simulink library "CRYP_OLSERVO"  (Simulink 8.6)
settings: Solver=VariableStepAuto  StartTime=0.0  StopTime=10.0  RelTol=1e-3
libraries: cdsTP x48, cdsEpicsOut x48, cdsFiltCtrl x25, cdsEpicsStringIn x24, cdsRms x24, cdsFilt x24, cdsMuxMatrix x2, lockin x1
(part 2 of 4)

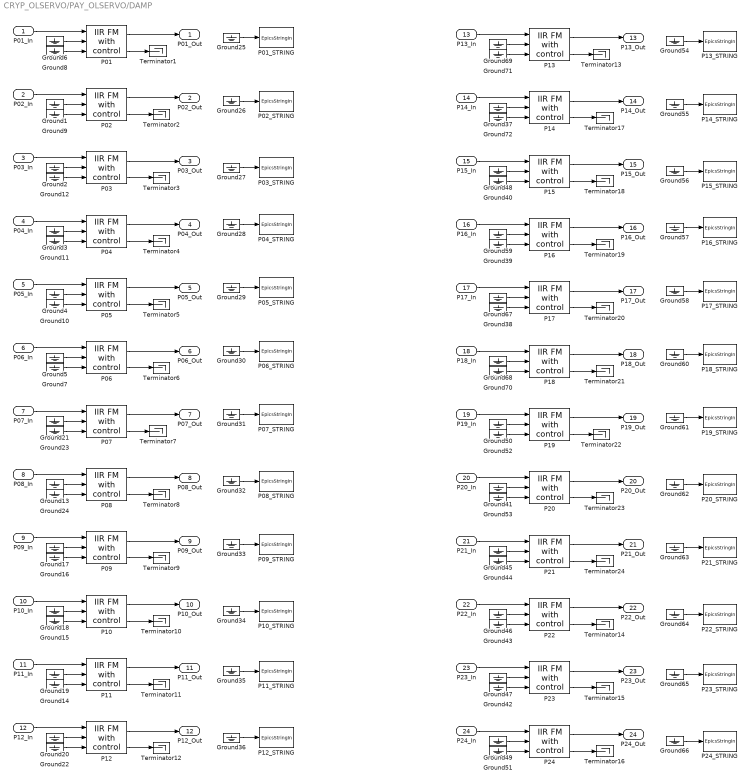
== system CRYP_OLSERVO/PAY_OLSERVO/DAMP ==
  P01_In : Inport
  P02_In : Inport  Port=2
  P03_In : Inport  Port=3
  P04_In : Inport  Port=4
  P05_In : Inport  Port=5
  P06_In : Inport  Port=6
  P07_In : Inport  Port=7
  P08_In : Inport  Port=8
  P09_In : Inport  Port=9
  P10_In : Inport  Port=10
  P11_In : Inport  Port=11
  P12_In : Inport  Port=12
  P13_In : Inport  Port=13
  P14_In : Inport  Port=14
  P15_In : Inport  Port=15
  P16_In : Inport  Port=16
  P17_In : Inport  Port=17
  P18_In : Inport  Port=18
  P19_In : Inport  Port=19
  P20_In : Inport  Port=20
  P21_In : Inport  Port=21
  P22_In : Inport  Port=22
  P23_In : Inport  Port=23
  P24_In : Inport  Port=24
  Ground{1..72} (72 alike) : Ground
  P01 : cdsFiltCtrl/IIR FM with control  Tag=cdsFiltCtrl  Description=|
      | cdsFiltCntrl is the standard IIR filter module (exactly the same as cdsFilt) but with added control data output 'Ctrl'. Filter module digital signal output appears on the first output, which is called 'Val'. 'Ctrl' output has a bit pattern encoding the state of filter's on/off switches (FM1 through FM10). The bit values are:
      |                                                                                                                                                                                                                                                                                                                                       
      | module 	hex	dec                                                                                                                                                                                                                                                                                                                       
      | -----------------------                                                                                                                                                                                                                                                                                                               
      | FM1	0x20                    32                                                                                                                                                                                                                                                                                                        
      | FM2	0x80                     128                                                                                                                                                                                                                                                                                                      
      | FM3	0x200                   512                                                                                                                                                                                                                                                                                                       
      | FM4	0x800                   2048                                                                                                                                                                                                                                                                                                      
      | FM5	0x2000                 8192                                                                                                                                                                                                                                                                                                       
      | FM6	0x8000                 32768                                                                                                                                                                                                                                                                                                      
      | FM7	0x20000                131072                                                                                                                                                                                                                                                                                                     
      | FM8	0x80000                 524288                                                                                                                                                                                                                                                                                                    
      | FM9	0x200000               2097152                                                                                                                                                                                                                                                                                                    
      | FM10	0x800000               8388608                                                                                                                                                                                                                                                                                                   
      |                                                                                                                                                                                                                                                                                                                                       
      | This bit data can be used to drive some other switches or it can be output using a binary I/O module.
      settings: AttributesFormatString=%<Tag>
  P01_STRING : cdsEpicsStringIn/EpicsStringIn  Tag=cdsEpicsStringIn  Description=cdsEpicsStringIn
      settings: AttributesFormatString=%<Tag>
  P02 : cdsFiltCtrl/IIR FM with control  Tag=cdsFiltCtrl  Description=|
      | cdsFiltCntrl is the standard IIR filter module (exactly the same as cdsFilt) but with added control data output 'Ctrl'. Filter module digital signal output appears on the first output, which is called 'Val'. 'Ctrl' output has a bit pattern encoding the state of filter's on/off switches (FM1 through FM10). The bit values are:
      |                                                                                                                                                                                                                                                                                                                                       
      | module 	hex	dec                                                                                                                                                                                                                                                                                                                       
      | -----------------------                                                                                                                                                                                                                                                                                                               
      | FM1	0x20                    32                                                                                                                                                                                                                                                                                                        
      | FM2	0x80                     128                                                                                                                                                                                                                                                                                                      
      | FM3	0x200                   512                                                                                                                                                                                                                                                                                                       
      | FM4	0x800                   2048                                                                                                                                                                                                                                                                                                      
      | FM5	0x2000                 8192                                                                                                                                                                                                                                                                                                       
      | FM6	0x8000                 32768                                                                                                                                                                                                                                                                                                      
      | FM7	0x20000                131072                                                                                                                                                                                                                                                                                                     
      | FM8	0x80000                 524288                                                                                                                                                                                                                                                                                                    
      | FM9	0x200000               2097152                                                                                                                                                                                                                                                                                                    
      | FM10	0x800000               8388608                                                                                                                                                                                                                                                                                                   
      |                                                                                                                                                                                                                                                                                                                                       
      | This bit data can be used to drive some other switches or it can be output using a binary I/O module.
      settings: AttributesFormatString=%<Tag>
  P02_STRING : cdsEpicsStringIn/EpicsStringIn  Tag=cdsEpicsStringIn  Description=cdsEpicsStringIn
      settings: AttributesFormatString=%<Tag>
  P03 : cdsFiltCtrl/IIR FM with control  Tag=cdsFiltCtrl  Description=|
      | cdsFiltCntrl is the standard IIR filter module (exactly the same as cdsFilt) but with added control data output 'Ctrl'. Filter module digital signal output appears on the first output, which is called 'Val'. 'Ctrl' output has a bit pattern encoding the state of filter's on/off switches (FM1 through FM10). The bit values are:
      |                                                                                                                                                                                                                                                                                                                                       
      | module 	hex	dec                                                                                                                                                                                                                                                                                                                       
      | -----------------------                                                                                                                                                                                                                                                                                                               
      | FM1	0x20                    32                                                                                                                                                                                                                                                                                                        
      | FM2	0x80                     128                                                                                                                                                                                                                                                                                                      
      | FM3	0x200                   512                                                                                                                                                                                                                                                                                                       
      | FM4	0x800                   2048                                                                                                                                                                                                                                                                                                      
      | FM5	0x2000                 8192                                                                                                                                                                                                                                                                                                       
      | FM6	0x8000                 32768                                                                                                                                                                                                                                                                                                      
      | FM7	0x20000                131072                                                                                                                                                                                                                                                                                                     
      | FM8	0x80000                 524288                                                                                                                                                                                                                                                                                                    
      | FM9	0x200000               2097152                                                                                                                                                                                                                                                                                                    
      | FM10	0x800000               8388608                                                                                                                                                                                                                                                                                                   
      |                                                                                                                                                                                                                                                                                                                                       
      | This bit data can be used to drive some other switches or it can be output using a binary I/O module.
      settings: AttributesFormatString=%<Tag>
  P03_STRING : cdsEpicsStringIn/EpicsStringIn  Tag=cdsEpicsStringIn  Description=cdsEpicsStringIn
      settings: AttributesFormatString=%<Tag>
  P04 : cdsFiltCtrl/IIR FM with control  Tag=cdsFiltCtrl  Description=|
      | cdsFiltCntrl is the standard IIR filter module (exactly the same as cdsFilt) but with added control data output 'Ctrl'. Filter module digital signal output appears on the first output, which is called 'Val'. 'Ctrl' output has a bit pattern encoding the state of filter's on/off switches (FM1 through FM10). The bit values are:
      |                                                                                                                                                                                                                                                                                                                                       
      | module 	hex	dec                                                                                                                                                                                                                                                                                                                       
      | -----------------------                                                                                                                                                                                                                                                                                                               
      | FM1	0x20                    32                                                                                                                                                                                                                                                                                                        
      | FM2	0x80                     128                                                                                                                                                                                                                                                                                                      
      | FM3	0x200                   512                                                                                                                                                                                                                                                                                                       
      | FM4	0x800                   2048                                                                                                                                                                                                                                                                                                      
      | FM5	0x2000                 8192                                                                                                                                                                                                                                                                                                       
      | FM6	0x8000                 32768                                                                                                                                                                                                                                                                                                      
      | FM7	0x20000                131072                                                                                                                                                                                                                                                                                                     
      | FM8	0x80000                 524288                                                                                                                                                                                                                                                                                                    
      | FM9	0x200000               2097152                                                                                                                                                                                                                                                                                                    
      | FM10	0x800000               8388608                                                                                                                                                                                                                                                                                                   
      |                                                                                                                                                                                                                                                                                                                                       
      | This bit data can be used to drive some other switches or it can be output using a binary I/O module.
      settings: AttributesFormatString=%<Tag>
  P04_STRING : cdsEpicsStringIn/EpicsStringIn  Tag=cdsEpicsStringIn  Description=cdsEpicsStringIn
      settings: AttributesFormatString=%<Tag>
  P05 : cdsFiltCtrl/IIR FM with control  Tag=cdsFiltCtrl  Description=|
      | cdsFiltCntrl is the standard IIR filter module (exactly the same as cdsFilt) but with added control data output 'Ctrl'. Filter module digital signal output appears on the first output, which is called 'Val'. 'Ctrl' output has a bit pattern encoding the state of filter's on/off switches (FM1 through FM10). The bit values are:
      |                                                                                                                                                                                                                                                                                                                                       
      | module 	hex	dec                                                                                                                                                                                                                                                                                                                       
      | -----------------------                                                                                                                                                                                                                                                                                                               
      | FM1	0x20                    32                                                                                                                                                                                                                                                                                                        
      | FM2	0x80                     128                                                                                                                                                                                                                                                                                                      
      | FM3	0x200                   512                                                                                                                                                                                                                                                                                                       
      | FM4	0x800                   2048                                                                                                                                                                                                                                                                                                      
      | FM5	0x2000                 8192                                                                                                                                                                                                                                                                                                       
      | FM6	0x8000                 32768                                                                                                                                                                                                                                                                                                      
      | FM7	0x20000                131072                                                                                                                                                                                                                                                                                                     
      | FM8	0x80000                 524288                                                                                                                                                                                                                                                                                                    
      | FM9	0x200000               2097152                                                                                                                                                                                                                                                                                                    
      | FM10	0x800000               8388608                                                                                                                                                                                                                                                                                                   
      |                                                                                                                                                                                                                                                                                                                                       
      | This bit data can be used to drive some other switches or it can be output using a binary I/O module.
      settings: AttributesFormatString=%<Tag>
  P05_STRING : cdsEpicsStringIn/EpicsStringIn  Tag=cdsEpicsStringIn  Description=cdsEpicsStringIn
      settings: AttributesFormatString=%<Tag>
  P06 : cdsFiltCtrl/IIR FM with control  Tag=cdsFiltCtrl  Description=|
      | cdsFiltCntrl is the standard IIR filter module (exactly the same as cdsFilt) but with added control data output 'Ctrl'. Filter module digital signal output appears on the first output, which is called 'Val'. 'Ctrl' output has a bit pattern encoding the state of filter's on/off switches (FM1 through FM10). The bit values are:
      |                                                                                                                                                                                                                                                                                                                                       
      | module 	hex	dec                                                                                                                                                                                                                                                                                                                       
      | -----------------------                                                                                                                                                                                                                                                                                                               
      | FM1	0x20                    32                                                                                                                                                                                                                                                                                                        
      | FM2	0x80                     128                                                                                                                                                                                                                                                                                                      
      | FM3	0x200                   512                                                                                                                                                                                                                                                                                                       
      | FM4	0x800                   2048                                                                                                                                                                                                                                                                                                      
      | FM5	0x2000                 8192                                                                                                                                                                                                                                                                                                       
      | FM6	0x8000                 32768                                                                                                                                                                                                                                                                                                      
      | FM7	0x20000                131072                                                                                                                                                                                                                                                                                                     
      | FM8	0x80000                 524288                                                                                                                                                                                                                                                                                                    
      | FM9	0x200000               2097152                                                                                                                                                                                                                                                                                                    
      | FM10	0x800000               8388608                                                                                                                                                                                                                                                                                                   
      |                                                                                                                                                                                                                                                                                                                                       
      | This bit data can be used to drive some other switches or it can be output using a binary I/O module.
      settings: AttributesFormatString=%<Tag>
  P06_STRING : cdsEpicsStringIn/EpicsStringIn  Tag=cdsEpicsStringIn  Description=cdsEpicsStringIn
      settings: AttributesFormatString=%<Tag>
  P07 : cdsFiltCtrl/IIR FM with control  Tag=cdsFiltCtrl  Description=|
      | cdsFiltCntrl is the standard IIR filter module (exactly the same as cdsFilt) but with added control data output 'Ctrl'. Filter module digital signal output appears on the first output, which is called 'Val'. 'Ctrl' output has a bit pattern encoding the state of filter's on/off switches (FM1 through FM10). The bit values are:
      |                                                                                                                                                                                                                                                                                                                                       
      | module 	hex	dec                                                                                                                                                                                                                                                                                                                       
      | -----------------------                                                                                                                                                                                                                                                                                                               
      | FM1	0x20                    32                                                                                                                                                                                                                                                                                                        
      | FM2	0x80                     128                                                                                                                                                                                                                                                                                                      
      | FM3	0x200                   512                                                                                                                                                                                                                                                                                                       
      | FM4	0x800                   2048                                                                                                                                                                                                                                                                                                      
      | FM5	0x2000                 8192                                                                                                                                                                                                                                                                                                       
      | FM6	0x8000                 32768                                                                                                                                                                                                                                                                                                      
      | FM7	0x20000                131072                                                                                                                                                                                                                                                                                                     
      | FM8	0x80000                 524288                                                                                                                                                                                                                                                                                                    
      | FM9	0x200000               2097152                                                                                                                                                                                                                                                                                                    
      | FM10	0x800000               8388608                                                                                                                                                                                                                                                                                                   
      |                                                                                                                                                                                                                                                                                                                                       
      | This bit data can be used to drive some other switches or it can be output using a binary I/O module.
      settings: AttributesFormatString=%<Tag>
  P07_STRING : cdsEpicsStringIn/EpicsStringIn  Tag=cdsEpicsStringIn  Description=cdsEpicsStringIn
      settings: AttributesFormatString=%<Tag>
  P08 : cdsFiltCtrl/IIR FM with control  Tag=cdsFiltCtrl  Description=|
      | cdsFiltCntrl is the standard IIR filter module (exactly the same as cdsFilt) but with added control data output 'Ctrl'. Filter module digital signal output appears on the first output, which is called 'Val'. 'Ctrl' output has a bit pattern encoding the state of filter's on/off switches (FM1 through FM10). The bit values are:
      |                                                                                                                                                                                                                                                                                                                                       
      | module 	hex	dec                                                                                                                                                                                                                                                                                                                       
      | -----------------------                                                                                                                                                                                                                                                                                                               
      | FM1	0x20                    32                                                                                                                                                                                                                                                                                                        
      | FM2	0x80                     128                                                                                                                                                                                                                                                                                                      
      | FM3	0x200                   512                                                                                                                                                                                                                                                                                                       
      | FM4	0x800                   2048                                                                                                                                                                                                                                                                                                      
      | FM5	0x2000                 8192                                                                                                                                                                                                                                                                                                       
      | FM6	0x8000                 32768                                                                                                                                                                                                                                                                                                      
      | FM7	0x20000                131072                                                                                                                                                                                                                                                                                                     
      | FM8	0x80000                 524288                                                                                                                                                                                                                                                                                                    
      | FM9	0x200000               2097152                                                                                                                                                                                                                                                                                                    
      | FM10	0x800000               8388608                                                                                                                                                                                                                                                                                                   
      |                                                                                                                                                                                                                                                                                                                                       
      | This bit data can be used to drive some other switches or it can be output using a binary I/O module.
      settings: AttributesFormatString=%<Tag>
  P08_STRING : cdsEpicsStringIn/EpicsStringIn  Tag=cdsEpicsStringIn  Description=cdsEpicsStringIn
      settings: AttributesFormatString=%<Tag>
  P09 : cdsFiltCtrl/IIR FM with control  Tag=cdsFiltCtrl  Description=|
      | cdsFiltCntrl is the standard IIR filter module (exactly the same as cdsFilt) but with added control data output 'Ctrl'. Filter module digital signal output appears on the first output, which is called 'Val'. 'Ctrl' output has a bit pattern encoding the state of filter's on/off switches (FM1 through FM10). The bit values are:
      |                                                                                                                                                                                                                                                                                                                                       
      | module 	hex	dec                                                                                                                                                                                                                                                                                                                       
      | -----------------------                                                                                                                                                                                                                                                                                                               
      | FM1	0x20                    32                                                                                                                                                                                                                                                                                                        
      | FM2	0x80                     128                                                                                                                                                                                                                                                                                                      
      | FM3	0x200                   512                                                                                                                                                                                                                                                                                                       
      | FM4	0x800                   2048                                                                                                                                                                                                                                                                                                      
      | FM5	0x2000                 8192                                                                                                                                                                                                                                                                                                       
      | FM6	0x8000                 32768                                                                                                                                                                                                                                                                                                      
      | FM7	0x20000                131072                                                                                                                                                                                                                                                                                                     
      | FM8	0x80000                 524288                                                                                                                                                                                                                                                                                                    
      | FM9	0x200000               2097152                                                                                                                                                                                                                                                                                                    
      | FM10	0x800000               8388608                                                                                                                                                                                                                                                                                                   
      |                                                                                                                                                                                                                                                                                                                                       
      | This bit data can be used to drive some other switches or it can be output using a binary I/O module.
      settings: AttributesFormatString=%<Tag>
  P09_STRING : cdsEpicsStringIn/EpicsStringIn  Tag=cdsEpicsStringIn  Description=cdsEpicsStringIn
      settings: AttributesFormatString=%<Tag>
  P10 : cdsFiltCtrl/IIR FM with control  Tag=cdsFiltCtrl  Description=|
      | cdsFiltCntrl is the standard IIR filter module (exactly the same as cdsFilt) but with added control data output 'Ctrl'. Filter module digital signal output appears on the first output, which is called 'Val'. 'Ctrl' output has a bit pattern encoding the state of filter's on/off switches (FM1 through FM10). The bit values are:
      |                                                                                                                                                                                                                                                                                                                                       
      | module 	hex	dec                                                                                                                                                                                                                                                                                                                       
      | -----------------------                                                                                                                                                                                                                                                                                                               
      | FM1	0x20                    32                                                                                                                                                                                                                                                                                                        
      | FM2	0x80                     128                                                                                                                                                                                                                                                                                                      
      | FM3	0x200                   512                                                                                                                                                                                                                                                                                                       
      | FM4	0x800                   2048                                                                                                                                                                                                                                                                                                      
      | FM5	0x2000                 8192                                                                                                                                                                                                                                                                                                       
      | FM6	0x8000                 32768                                                                                                                                                                                                                                                                                                      
      | FM7	0x20000                131072                                                                                                                                                                                                                                                                                                     
      | FM8	0x80000                 524288                                                                                                                                                                                                                                                                                                    
      | FM9	0x200000               2097152                                                                                                                                                                                                                                                                                                    
      | FM10	0x800000               8388608                                                                                                                                                                                                                                                                                                   
      |                                                                                                                                                                                                                                                                                                                                       
      | This bit data can be used to drive some other switches or it can be output using a binary I/O module.
      settings: AttributesFormatString=%<Tag>
  P10_STRING : cdsEpicsStringIn/EpicsStringIn  Tag=cdsEpicsStringIn  Description=cdsEpicsStringIn
      settings: AttributesFormatString=%<Tag>
  P11 : cdsFiltCtrl/IIR FM with control  Tag=cdsFiltCtrl  Description=|
      | cdsFiltCntrl is the standard IIR filter module (exactly the same as cdsFilt) but with added control data output 'Ctrl'. Filter module digital signal output appears on the first output, which is called 'Val'. 'Ctrl' output has a bit pattern encoding the state of filter's on/off switches (FM1 through FM10). The bit values are:
      |                                                                                                                                                                                                                                                                                                                                       
      | module 	hex	dec                                                                                                                                                                                                                                                                                                                       
      | -----------------------                                                                                                                                                                                                                                                                                                               
      | FM1	0x20                    32                                                                                                                                                                                                                                                                                                        
      | FM2	0x80                     128                                                                                                                                                                                                                                                                                                      
      | FM3	0x200                   512                                                                                                                                                                                                                                                                                                       
      | FM4	0x800                   2048                                                                                                                                                                                                                                                                                                      
      | FM5	0x2000                 8192                                                                                                                                                                                                                                                                                                       
      | FM6	0x8000                 32768                                                                                                                                                                                                                                                                                                      
      | FM7	0x20000                131072                                                                                                                                                                                                                                                                                                     
      | FM8	0x80000                 524288                                                                                                                                                                                                                                                                                                    
      | FM9	0x200000               2097152                                                                                                                                                                                                                                                                                                    
      | FM10	0x800000               8388608                                                                                                                                                                                                                                                                                                   
      |                                                                                                                                                                                                                                                                                                                                       
      | This bit data can be used to drive some other switches or it can be output using a binary I/O module.
      settings: AttributesFormatString=%<Tag>
  P11_STRING : cdsEpicsStringIn/EpicsStringIn  Tag=cdsEpicsStringIn  Description=cdsEpicsStringIn
      settings: AttributesFormatString=%<Tag>
  P12 : cdsFiltCtrl/IIR FM with control  Tag=cdsFiltCtrl  Description=|
      | cdsFiltCntrl is the standard IIR filter module (exactly the same as cdsFilt) but with added control data output 'Ctrl'. Filter module digital signal output appears on the first output, which is called 'Val'. 'Ctrl' output has a bit pattern encoding the state of filter's on/off switches (FM1 through FM10). The bit values are:
      |                                                                                                                                                                                                                                                                                                                                       
      | module 	hex	dec                                                                                                                                                                                                                                                                                                                       
      | -----------------------                                                                                                                                                                                                                                                                                                               
      | FM1	0x20                    32                                                                                                                                                                                                                                                                                                        
      | FM2	0x80                     128                                                                                                                                                                                                                                                                                                      
      | FM3	0x200                   512                                                                                                                                                                                                                                                                                                       
      | FM4	0x800                   2048                                                                                                                                                                                                                                                                                                      
      | FM5	0x2000                 8192                                                                                                                                                                                                                                                                                                       
      | FM6	0x8000                 32768                                                                                                                                                                                                                                                                                                      
      | FM7	0x20000                131072                                                                                                                                                                                                                                                                                                     
      | FM8	0x80000                 524288                                                                                                                                                                                                                                                                                                    
      | FM9	0x200000               2097152                                                                                                                                                                                                                                                                                                    
      | FM10	0x800000               8388608                                                                                                                                                                                                                                                                                                   
      |                                                                                                                                                                                                                                                                                                                                       
      | This bit data can be used to drive some other switches or it can be output using a binary I/O module.
      settings: AttributesFormatString=%<Tag>
  P12_STRING : cdsEpicsStringIn/EpicsStringIn  Tag=cdsEpicsStringIn  Description=cdsEpicsStringIn
      settings: AttributesFormatString=%<Tag>
  P13 : cdsFiltCtrl/IIR FM with control  Tag=cdsFiltCtrl  Description=|
      | cdsFiltCntrl is the standard IIR filter module (exactly the same as cdsFilt) but with added control data output 'Ctrl'. Filter module digital signal output appears on the first output, which is called 'Val'. 'Ctrl' output has a bit pattern encoding the state of filter's on/off switches (FM1 through FM10). The bit values are:
      |                                                                                                                                                                                                                                                                                                                                       
      | module 	hex	dec                                                                                                                                                                                                                                                                                                                       
      | -----------------------                                                                                                                                                                                                                                                                                                               
      | FM1	0x20                    32                                                                                                                                                                                                                                                                                                        
      | FM2	0x80                     128                                                                                                                                                                                                                                                                                                      
      | FM3	0x200                   512                                                                                                                                                                                                                                                                                                       
      | FM4	0x800                   2048                                                                                                                                                                                                                                                                                                      
      | FM5	0x2000                 8192                                                                                                                                                                                                                                                                                                       
      | FM6	0x8000                 32768                                                                                                                                                                                                                                                                                                      
      | FM7	0x20000                131072                                                                                                                                                                                                                                                                                                     
      | FM8	0x80000                 524288                                                                                                                                                                                                                                                                                                    
      | FM9	0x200000               2097152                                                                                                                                                                                                                                                                                                    
      | FM10	0x800000               8388608                                                                                                                                                                                                                                                                                                   
      |                                                                                                                                                                                                                                                                                                                                       
      | This bit data can be used to drive some other switches or it can be output using a binary I/O module.
      settings: AttributesFormatString=%<Tag>
  P13_STRING : cdsEpicsStringIn/EpicsStringIn  Tag=cdsEpicsStringIn  Description=cdsEpicsStringIn
      settings: AttributesFormatString=%<Tag>
  P14 : cdsFiltCtrl/IIR FM with control  Tag=cdsFiltCtrl  Description=|
      | cdsFiltCntrl is the standard IIR filter module (exactly the same as cdsFilt) but with added control data output 'Ctrl'. Filter module digital signal output appears on the first output, which is called 'Val'. 'Ctrl' output has a bit pattern encoding the state of filter's on/off switches (FM1 through FM10). The bit values are:
      |                                                                                                                                                                                                                                                                                                                                       
      | module 	hex	dec                                                                                                                                                                                                                                                                                                                       
      | -----------------------                                                                                                                                                                                                                                                                                                               
      | FM1	0x20                    32                                                                                                                                                                                                                                                                                                        
      | FM2	0x80                     128                                                                                                                                                                                                                                                                                                      
      | FM3	0x200                   512                                                                                                                                                                                                                                                                                                       
      | FM4	0x800                   2048                                                                                                                                                                                                                                                                                                      
      | FM5	0x2000                 8192                                                                                                                                                                                                                                                                                                       
      | FM6	0x8000                 32768                                                                                                                                                                                                                                                                                                      
      | FM7	0x20000                131072                                                                                                                                                                                                                                                                                                     
      | FM8	0x80000                 524288                                                                                                                                                                                                                                                                                                    
      | FM9	0x200000               2097152                                                                                                                                                                                                                                                                                                    
      | FM10	0x800000               8388608                                                                                                                                                                                                                                                                                                   
      |                                                                                                                                                                                                                                                                                                                                       
      | This bit data can be used to drive some other switches or it can be output using a binary I/O module.
      settings: AttributesFormatString=%<Tag>
  P14_STRING : cdsEpicsStringIn/EpicsStringIn  Tag=cdsEpicsStringIn  Description=cdsEpicsStringIn
      settings: AttributesFormatString=%<Tag>
  P15 : cdsFiltCtrl/IIR FM with control  Tag=cdsFiltCtrl  Description=|
      | cdsFiltCntrl is the standard IIR filter module (exactly the same as cdsFilt) but with added control data output 'Ctrl'. Filter module digital signal output appears on the first output, which is called 'Val'. 'Ctrl' output has a bit pattern encoding the state of filter's on/off switches (FM1 through FM10). The bit values are:
      |                                                                                                                                                                                                                                                                                                                                       
      | module 	hex	dec                                                                                                                                                                                                                                                                                                                       
      | -----------------------                                                                                                                                                                                                                                                                                                               
      | FM1	0x20                    32                                                                                                                                                                                                                                                                                                        
      | FM2	0x80                     128                                                                                                                                                                                                                                                                                                      
      | FM3	0x200                   512                                                                                                                                                                                                                                                                                                       
      | FM4	0x800                   2048                                                                                                                                                                                                                                                                                                      
      | FM5	0x2000                 8192                                                                                                                                                                                                                                                                                                       
      | FM6	0x8000                 32768                                                                                                                                                                                                                                                                                                      
      | FM7	0x20000                131072                                                                                                                                                                                                                                                                                                     
      | FM8	0x80000                 524288                                                                                                                                                                                                                                                                                                    
      | FM9	0x200000               2097152                                                                                                                                                                                                                                                                                                    
      | FM10	0x800000               8388608                                                                                                                                                                                                                                                                                                   
      |                                                                                                                                                                                                                                                                                                                                       
      | This bit data can be used to drive some other switches or it can be output using a binary I/O module.
      settings: AttributesFormatString=%<Tag>
  P15_STRING : cdsEpicsStringIn/EpicsStringIn  Tag=cdsEpicsStringIn  Description=cdsEpicsStringIn
      settings: AttributesFormatString=%<Tag>
  P16 : cdsFiltCtrl/IIR FM with control  Tag=cdsFiltCtrl  Description=|
      | cdsFiltCntrl is the standard IIR filter module (exactly the same as cdsFilt) but with added control data output 'Ctrl'. Filter module digital signal output appears on the first output, which is called 'Val'. 'Ctrl' output has a bit pattern encoding the state of filter's on/off switches (FM1 through FM10). The bit values are:
      |                                                                                                                                                                                                                                                                                                                                       
      | module 	hex	dec                                                                                                                                                                                                                                                                                                                       
      | -----------------------                                                                                                                                                                                                                                                                                                               
      | FM1	0x20                    32                                                                                                                                                                                                                                                                                                        
      | FM2	0x80                     128                                                                                                                                                                                                                                                                                                      
      | FM3	0x200                   512                                                                                                                                                                                                                                                                                                       
      | FM4	0x800                   2048                                                                                                                                                                                                                                                                                                      
      | FM5	0x2000                 8192                                                                                                                                                                                                                                                                                                       
      | FM6	0x8000                 32768                                                                                                                                                                                                                                                                                                      
      | FM7	0x20000                131072                                                                                                                                                                                                                                                                                                     
      | FM8	0x80000                 524288                                                                                                                                                                                                                                                                                                    
      | FM9	0x200000               2097152                                                                                                                                                                                                                                                                                                    
      | FM10	0x800000               8388608                                                                                                                                                                                                                                                                                                   
      |                                                                                                                                                                                                                                                                                                                                       
      | This bit data can be used to drive some other switches or it can be output using a binary I/O module.
      settings: AttributesFormatString=%<Tag>
  P16_STRING : cdsEpicsStringIn/EpicsStringIn  Tag=cdsEpicsStringIn  Description=cdsEpicsStringIn
      settings: AttributesFormatString=%<Tag>
  P17 : cdsFiltCtrl/IIR FM with control  Tag=cdsFiltCtrl  Description=|
      | cdsFiltCntrl is the standard IIR filter module (exactly the same as cdsFilt) but with added control data output 'Ctrl'. Filter module digital signal output appears on the first output, which is called 'Val'. 'Ctrl' output has a bit pattern encoding the state of filter's on/off switches (FM1 through FM10). The bit values are:
      |                                                                                                                                                                                                                                                                                                                                       
      | module 	hex	dec                                                                                                                                                                                                                                                                                                                       
      | -----------------------                                                                                                                                                                                                                                                                                                               
      | FM1	0x20                    32                                                                                                                                                                                                                                                                                                        
      | FM2	0x80                     128                                                                                                                                                                                                                                                                                                      
      | FM3	0x200                   512                                                                                                                                                                                                                                                                                                       
      | FM4	0x800                   2048                                                                                                                                                                                                                                                                                                      
      | FM5	0x2000                 8192                                                                                                                                                                                                                                                                                                       
      | FM6	0x8000                 32768                                                                                                                                                                                                                                                                                                      
      | FM7	0x20000                131072                                                                                                                                                                                                                                                                                                     
      | FM8	0x80000                 524288                                                                                                                                                                                                                                                                                                    
      | FM9	0x200000               2097152                                                                                                                                                                                                                                                                                                    
      | FM10	0x800000               8388608                                                                                                                                                                                                                                                                                                   
      |                                                                                                                                                                                                                                                                                                                                       
      | This bit data can be used to drive some other switches or it can be output using a binary I/O module.
      settings: AttributesFormatString=%<Tag>
  P17_STRING : cdsEpicsStringIn/EpicsStringIn  Tag=cdsEpicsStringIn  Description=cdsEpicsStringIn
      settings: AttributesFormatString=%<Tag>
  P18 : cdsFiltCtrl/IIR FM with control  Tag=cdsFiltCtrl  Description=|
      | cdsFiltCntrl is the standard IIR filter module (exactly the same as cdsFilt) but with added control data output 'Ctrl'. Filter module digital signal output appears on the first output, which is called 'Val'. 'Ctrl' output has a bit pattern encoding the state of filter's on/off switches (FM1 through FM10). The bit values are:
      |                                                                                                                                                                                                                                                                                                                                       
      | module 	hex	dec                                                                                                                                                                                                                                                                                                                       
      | -----------------------                                                                                                                                                                                                                                                                                                               
      | FM1	0x20                    32                                                                                                                                                                                                                                                                                                        
      | FM2	0x80                     128                                                                                                                                                                                                                                                                                                      
      | FM3	0x200                   512                                                                                                                                                                                                                                                                                                       
      | FM4	0x800                   2048                                                                                                                                                                                                                                                                                                      
      | FM5	0x2000                 8192                                                                                                                                                                                                                                                                                                       
      | FM6	0x8000                 32768                                                                                                                                                                                                                                                                                                      
      | FM7	0x20000                131072                                                                                                                                                                                                                                                                                                     
      | FM8	0x80000                 524288                                                                                                                                                                                                                                                                                                    
      | FM9	0x200000               2097152                                                                                                                                                                                                                                                                                                    
      | FM10	0x800000               8388608                                                                                                                                                                                                                                                                                                   
      |                                                                                                                                                                                                                                                                                                                                       
      | This bit data can be used to drive some other switches or it can be output using a binary I/O module.
      settings: AttributesFormatString=%<Tag>
  P18_STRING : cdsEpicsStringIn/EpicsStringIn  Tag=cdsEpicsStringIn  Description=cdsEpicsStringIn
      settings: AttributesFormatString=%<Tag>
  P19 : cdsFiltCtrl/IIR FM with control  Tag=cdsFiltCtrl  Description=|
      | cdsFiltCntrl is the standard IIR filter module (exactly the same as cdsFilt) but with added control data output 'Ctrl'. Filter module digital signal output appears on the first output, which is called 'Val'. 'Ctrl' output has a bit pattern encoding the state of filter's on/off switches (FM1 through FM10). The bit values are:
      |                                                                                                                                                                                                                                                                                                                                       
      | module 	hex	dec                                                                                                                                                                                                                                                                                                                       
      | -----------------------                                                                                                                                                                                                                                                                                                               
      | FM1	0x20                    32                                                                                                                                                                                                                                                                                                        
      | FM2	0x80                     128                                                                                                                                                                                                                                                                                                      
      | FM3	0x200                   512                                                                                                                                                                                                                                                                                                       
      | FM4	0x800                   2048                                                                                                                                                                                                                                                                                                      
      | FM5	0x2000                 8192                                                                                                                                                                                                                                                                                                       
      | FM6	0x8000                 32768                                                                                                                                                                                                                                                                                                      
      | FM7	0x20000                131072                                                                                                                                                                                                                                                                                                     
      | FM8	0x80000                 524288                                                                                                                                                                                                                                                                                                    
      | FM9	0x200000               2097152                                                                                                                                                                                                                                                                                                    
      | FM10	0x800000               8388608                                                                                                                                                                                                                                                                                                   
      |                                                                                                                                                                                                                                                                                                                                       
      | This bit data can be used to drive some other switches or it can be output using a binary I/O module.
      settings: AttributesFormatString=%<Tag>
  P19_STRING : cdsEpicsStringIn/EpicsStringIn  Tag=cdsEpicsStringIn  Description=cdsEpicsStringIn
      settings: AttributesFormatString=%<Tag>
  P20 : cdsFiltCtrl/IIR FM with control  Tag=cdsFiltCtrl  Description=|
      | cdsFiltCntrl is the standard IIR filter module (exactly the same as cdsFilt) but with added control data output 'Ctrl'. Filter module digital signal output appears on the first output, which is called 'Val'. 'Ctrl' output has a bit pattern encoding the state of filter's on/off switches (FM1 through FM10). The bit values are:
      |                                                                                                                                                                                                                                                                                                                                       
      | module 	hex	dec                                                                                                                                                                                                                                                                                                                       
      | -----------------------                                                                                                                                                                                                                                                                                                               
      | FM1	0x20                    32                                                                                                                                                                                                                                                                                                        
      | FM2	0x80                     128                                                                                                                                                                                                                                                                                                      
      | FM3	0x200                   512                                                                                                                                                                                                                                                                                                       
      | FM4	0x800                   2048                                                                                                                                                                                                                                                                                                      
      | FM5	0x2000                 8192                                                                                                                                                                                                                                                                                                       
      | FM6	0x8000                 32768                                                                                                                                                                                                                                                                                                      
      | FM7	0x20000                131072                                                                                                                                                                                                                                                                                                     
      | FM8	0x80000                 524288                                                                                                                                                                                                                                                                                                    
      | FM9	0x200000               2097152                                                                                                                                                                                                                                                                                                    
      | FM10	0x800000               8388608                                                                                                                                                                                                                                                                                                   
      |                                                                                                                                                                                                                                                                                                                                       
      | This bit data can be used to drive some other switches or it can be output using a binary I/O module.
      settings: AttributesFormatString=%<Tag>
  P20_STRING : cdsEpicsStringIn/EpicsStringIn  Tag=cdsEpicsStringIn  Description=cdsEpicsStringIn
      settings: AttributesFormatString=%<Tag>
  P21 : cdsFiltCtrl/IIR FM with control  Tag=cdsFiltCtrl  Description=|
      | cdsFiltCntrl is the standard IIR filter module (exactly the same as cdsFilt) but with added control data output 'Ctrl'. Filter module digital signal output appears on the first output, which is called 'Val'. 'Ctrl' output has a bit pattern encoding the state of filter's on/off switches (FM1 through FM10). The bit values are:
      |                                                                                                                                                                                                                                                                                                                                       
      | module 	hex	dec                                                                                                                                                                                                                                                                                                                       
      | -----------------------                                                                                                                                                                                                                                                                                                               
      | FM1	0x20                    32                                                                                                                                                                                                                                                                                                        
      | FM2	0x80                     128                                                                                                                                                                                                                                                                                                      
      | FM3	0x200                   512                                                                                                                                                                                                                                                                                                       
      | FM4	0x800                   2048                                                                                                                                                                                                                                                                                                      
      | FM5	0x2000                 8192                                                                                                                                                                                                                                                                                                       
      | FM6	0x8000                 32768                                                                                                                                                                                                                                                                                                      
      | FM7	0x20000                131072                                                                                                                                                                                                                                                                                                     
      | FM8	0x80000                 524288                                                                                                                                                                                                                                                                                                    
      | FM9	0x200000               2097152                                                                                                                                                                                                                                                                                                    
      | FM10	0x800000               8388608                                                                                                                                                                                                                                                                                                   
      |                                                                                                                                                                                                                                                                                                                                       
      | This bit data can be used to drive some other switches or it can be output using a binary I/O module.
      settings: AttributesFormatString=%<Tag>
  P21_STRING : cdsEpicsStringIn/EpicsStringIn  Tag=cdsEpicsStringIn  Description=cdsEpicsStringIn
      settings: AttributesFormatString=%<Tag>
  P22 : cdsFiltCtrl/IIR FM with control  Tag=cdsFiltCtrl  Description=|
      | cdsFiltCntrl is the standard IIR filter module (exactly the same as cdsFilt) but with added control data output 'Ctrl'. Filter module digital signal output appears on the first output, which is called 'Val'. 'Ctrl' output has a bit pattern encoding the state of filter's on/off switches (FM1 through FM10). The bit values are:
      |                                                                                                                                                                                                                                                                                                                                       
      | module 	hex	dec                                                                                                                                                                                                                                                                                                                       
      | -----------------------                                                                                                                                                                                                                                                                                                               
      | FM1	0x20                    32                                                                                                                                                                                                                                                                                                        
      | FM2	0x80                     128                                                                                                                                                                                                                                                                                                      
      | FM3	0x200                   512                                                                                                                                                                                                                                                                                                       
      | FM4	0x800                   2048                                                                                                                                                                                                                                                                                                      
      | FM5	0x2000                 8192                                                                                                                                                                                                                                                                                                       
      | FM6	0x8000                 32768                                                                                                                                                                                                                                                                                                      
      | FM7	0x20000                131072                                                                                                                                                                                                                                                                                                     
      | FM8	0x80000                 524288                                                                                                                                                                                                                                                                                                    
      | FM9	0x200000               2097152                                                                                                                                                                                                                                                                                                    
      | FM10	0x800000               8388608                                                                                                                                                                                                                                                                                                   
      |                                                                                                                                                                                                                                                                                                                                       
      | This bit data can be used to drive some other switches or it can be output using a binary I/O module.
      settings: AttributesFormatString=%<Tag>
  P22_STRING : cdsEpicsStringIn/EpicsStringIn  Tag=cdsEpicsStringIn  Description=cdsEpicsStringIn
      settings: AttributesFormatString=%<Tag>
  P23 : cdsFiltCtrl/IIR FM with control  Tag=cdsFiltCtrl  Description=|
      | cdsFiltCntrl is the standard IIR filter module (exactly the same as cdsFilt) but with added control data output 'Ctrl'. Filter module digital signal output appears on the first output, which is called 'Val'. 'Ctrl' output has a bit pattern encoding the state of filter's on/off switches (FM1 through FM10). The bit values are:
      |                                                                                                                                                                                                                                                                                                                                       
      | module 	hex	dec                                                                                                                                                                                                                                                                                                                       
      | -----------------------                                                                                                                                                                                                                                                                                                               
      | FM1	0x20                    32                                                                                                                                                                                                                                                                                                        
      | FM2	0x80                     128                                                                                                                                                                                                                                                                                                      
      | FM3	0x200                   512                                                                                                                                                                                                                                                                                                       
      | FM4	0x800                   2048                                                                                                                                                                                                                                                                                                      
      | FM5	0x2000                 8192                                                                                                                                                                                                                                                                                                       
      | FM6	0x8000                 32768                                                                                                                                                                                                                                                                                                      
      | FM7	0x20000                131072                                                                                                                                                                                                                                                                                                     
      | FM8	0x80000                 524288                                                                                                                                                                                                                                                                                                    
      | FM9	0x200000               2097152                                                                                                                                                                                                                                                                                                    
      | FM10	0x800000               8388608                                                                                                                                                                                                                                                                                                   
      |                                                                                                                                                                                                                                                                                                                                       
      | This bit data can be used to drive some other switches or it can be output using a binary I/O module.
      settings: AttributesFormatString=%<Tag>
  P23_STRING : cdsEpicsStringIn/EpicsStringIn  Tag=cdsEpicsStringIn  Description=cdsEpicsStringIn
      settings: AttributesFormatString=%<Tag>
  P24 : cdsFiltCtrl/IIR FM with control  Tag=cdsFiltCtrl  Description=|
      | cdsFiltCntrl is the standard IIR filter module (exactly the same as cdsFilt) but with added control data output 'Ctrl'. Filter module digital signal output appears on the first output, which is called 'Val'. 'Ctrl' output has a bit pattern encoding the state of filter's on/off switches (FM1 through FM10). The bit values are:
      |                                                                                                                                                                                                                                                                                                                                       
      | module 	hex	dec                                                                                                                                                                                                                                                                                                                       
      | -----------------------                                                                                                                                                                                                                                                                                                               
      | FM1	0x20                    32                                                                                                                                                                                                                                                                                                        
      | FM2	0x80                     128                                                                                                                                                                                                                                                                                                      
      | FM3	0x200                   512                                                                                                                                                                                                                                                                                                       
      | FM4	0x800                   2048                                                                                                                                                                                                                                                                                                      
      | FM5	0x2000                 8192                                                                                                                                                                                                                                                                                                       
      | FM6	0x8000                 32768                                                                                                                                                                                                                                                                                                      
      | FM7	0x20000                131072                                                                                                                                                                                                                                                                                                     
      | FM8	0x80000                 524288                                                                                                                                                                                                                                                                                                    
      | FM9	0x200000               2097152                                                                                                                                                                                                                                                                                                    
      | FM10	0x800000               8388608                                                                                                                                                                                                                                                                                                   
      |                                                                                                                                                                                                                                                                                                                                       
      | This bit data can be used to drive some other switches or it can be output using a binary I/O module.
      settings: AttributesFormatString=%<Tag>
  P24_STRING : cdsEpicsStringIn/EpicsStringIn  Tag=cdsEpicsStringIn  Description=cdsEpicsStringIn
      settings: AttributesFormatString=%<Tag>
  Terminator{1..24} (24 alike) : Terminator
  P01_Out : Outport
  P02_Out : Outport  Port=2
  P03_Out : Outport  Port=3
  P04_Out : Outport  Port=4
  P05_Out : Outport  Port=5
  P06_Out : Outport  Port=6
  P07_Out : Outport  Port=7
  P08_Out : Outport  Port=8
  P09_Out : Outport  Port=9
  P10_Out : Outport  Port=10
  P11_Out : Outport  Port=11
  P12_Out : Outport  Port=12
  P13_Out : Outport  Port=13
  P14_Out : Outport  Port=14
  P15_Out : Outport  Port=15
  P16_Out : Outport  Port=16
  P17_Out : Outport  Port=17
  P18_Out : Outport  Port=18
  P19_Out : Outport  Port=19
  P20_Out : Outport  Port=20
  P21_Out : Outport  Port=21
  P22_Out : Outport  Port=22
  P23_Out : Outport  Port=23
  P24_Out : Outport  Port=24
  wires:
  Ground12/1 -> P03/3
  Ground11/1 -> P04/3
  Ground10/1 -> P05/3
  Ground9/1 -> P02/3
  Ground8/1 -> P01/3
  Ground7/1 -> P06/3
  P02_In/1 -> P02/1
  P03_In/1 -> P03/1
  P04_In/1 -> P04/1
  P05_In/1 -> P05/1
  P02/1 -> P02_Out/1
  P03/1 -> P03_Out/1
  P06_In/1 -> P06/1
  P01/1 -> P01_Out/1
  P01_In/1 -> P01/1
  Ground5/1 -> P06/2
  Ground4/1 -> P05/2
  Ground3/1 -> P04/2
  Ground2/1 -> P03/2
  Ground1/1 -> P02/2
  Ground6/1 -> P01/2
  P06/1 -> P06_Out/1
  P05/1 -> P05_Out/1
  P04/1 -> P04_Out/1
  P01/2 -> Terminator1/1
  P02/2 -> Terminator2/1
  P03/2 -> Terminator3/1
  P04/2 -> Terminator4/1
  P05/2 -> Terminator5/1
  P06/2 -> Terminator6/1
  Ground16/1 -> P09/3
  Ground15/1 -> P10/3
  Ground14/1 -> P11/3
  Ground24/1 -> P08/3
  Ground23/1 -> P07/3
  Ground22/1 -> P12/3
  P08_In/1 -> P08/1
  P09_In/1 -> P09/1
  P10_In/1 -> P10/1
  P11_In/1 -> P11/1
  P08/1 -> P08_Out/1
  P09/1 -> P09_Out/1
  P12_In/1 -> P12/1
  P07/1 -> P07_Out/1
  P07_In/1 -> P07/1
  Ground20/1 -> P12/2
  Ground19/1 -> P11/2
  Ground18/1 -> P10/2
  Ground17/1 -> P09/2
  Ground13/1 -> P08/2
  Ground21/1 -> P07/2
  P12/1 -> P12_Out/1
  P11/1 -> P11_Out/1
  P10/1 -> P10_Out/1
  P07/2 -> Terminator7/1
  P08/2 -> Terminator8/1
  P09/2 -> Terminator9/1
  P10/2 -> Terminator10/1
  P11/2 -> Terminator11/1
  P12/2 -> Terminator12/1
  Ground25/1 -> P01_STRING/1
  Ground26/1 -> P02_STRING/1
  Ground27/1 -> P03_STRING/1
  Ground28/1 -> P04_STRING/1
  Ground29/1 -> P05_STRING/1
  Ground30/1 -> P06_STRING/1
  Ground31/1 -> P07_STRING/1
  Ground32/1 -> P08_STRING/1
  Ground33/1 -> P09_STRING/1
  Ground34/1 -> P10_STRING/1
  Ground35/1 -> P11_STRING/1
  Ground36/1 -> P12_STRING/1
  Ground40/1 -> P15/3
  Ground39/1 -> P16/3
  Ground38/1 -> P17/3
  Ground72/1 -> P14/3
  Ground71/1 -> P13/3
  Ground70/1 -> P18/3
  P14_In/1 -> P14/1
  P15_In/1 -> P15/1
  P16_In/1 -> P16/1
  P17_In/1 -> P17/1
  P14/1 -> P14_Out/1
  P15/1 -> P15_Out/1
  P18_In/1 -> P18/1
  P13/1 -> P13_Out/1
  P13_In/1 -> P13/1
  Ground68/1 -> P18/2
  Ground67/1 -> P17/2
  Ground59/1 -> P16/2
  Ground48/1 -> P15/2
  Ground37/1 -> P14/2
  Ground69/1 -> P13/2
  P18/1 -> P18_Out/1
  P17/1 -> P17_Out/1
  P16/1 -> P16_Out/1
  P13/2 -> Terminator13/1
  P14/2 -> Terminator17/1
  P15/2 -> Terminator18/1
  P16/2 -> Terminator19/1
  P17/2 -> Terminator20/1
  P18/2 -> Terminator21/1
  Ground44/1 -> P21/3
  Ground43/1 -> P22/3
  Ground42/1 -> P23/3
  Ground53/1 -> P20/3
  Ground52/1 -> P19/3
  Ground51/1 -> P24/3
  P20_In/1 -> P20/1
  P21_In/1 -> P21/1
  P22_In/1 -> P22/1
  P23_In/1 -> P23/1
  P20/1 -> P20_Out/1
  P21/1 -> P21_Out/1
  P24_In/1 -> P24/1
  P19/1 -> P19_Out/1
  P19_In/1 -> P19/1
  Ground49/1 -> P24/2
  Ground47/1 -> P23/2
  Ground46/1 -> P22/2
  Ground45/1 -> P21/2
  Ground41/1 -> P20/2
  Ground50/1 -> P19/2
  P24/1 -> P24_Out/1
  P23/1 -> P23_Out/1
  P22/1 -> P22_Out/1
  P19/2 -> Terminator22/1
  P20/2 -> Terminator23/1
  P21/2 -> Terminator24/1
  P22/2 -> Terminator14/1
  P23/2 -> Terminator15/1
  P24/2 -> Terminator16/1
  Ground54/1 -> P13_STRING/1
  Ground55/1 -> P14_STRING/1
  Ground56/1 -> P15_STRING/1
  Ground57/1 -> P16_STRING/1
  Ground58/1 -> P17_STRING/1
  Ground60/1 -> P18_STRING/1
  Ground61/1 -> P19_STRING/1
  Ground62/1 -> P20_STRING/1
  Ground63/1 -> P21_STRING/1
  Ground64/1 -> P22_STRING/1
  Ground65/1 -> P23_STRING/1
  Ground66/1 -> P24_STRING/1
